simulink model "ProposedProblem5"  (R2013a)
settings: Solver=ode45  StartTime=0.0  StopTime=3600  RelTol=1e-3
undefined symbols (not defined in the file): des, gcbh
settings Model: Creator=gabig  LastModifiedBy=gabig

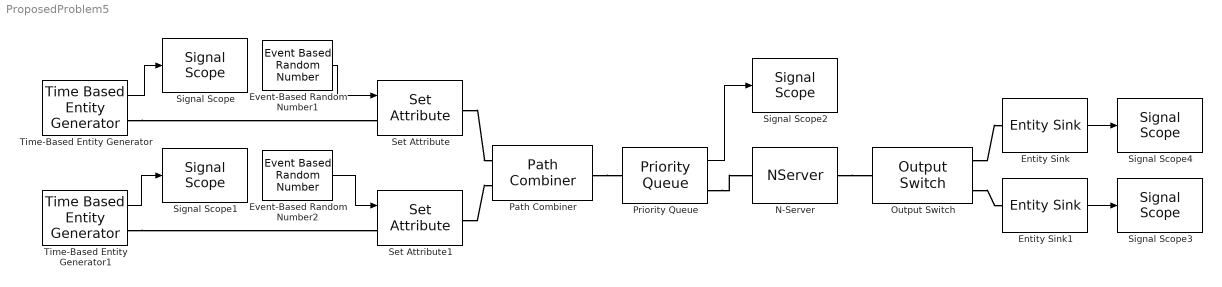
== system ProposedProblem5 ==
  Entity Sink : EntitySink  StatNumberArrived=on
  Entity Sink1 : EntitySink  StatNumberArrived=on
  Event-Based Random Number1 : EventBasedRandomNumber  Distribution=Uniform  minUnif=21  maxUnif=39  Seed=12321
  Event-Based Random Number2 : EventBasedRandomNumber  Distribution=Uniform  minUnif=9  maxUnif=15  Seed=12312
  N-Server : NServer  NumberOfServers=2  ServiceTimeFrom=Attribute  AttributeName=WORKER
  Output Switch : OutputSwitch  NumberOutputPorts=2  SwitchingCriterion=From attribute  AttributeName=p1
  Path Combiner : PathCombiner  NumberInputPorts=2
  Priority Queue : PriorityQueue  SortingAttributeName=p1  SortingDirection=Descending  StatAverageQueueLength=on
      settings: OutputPortMap=o3
  Set Attribute : SetAttribute  AttributeName=WORKER|p1  AttributeFrom=Signal port|Dialog  AttributeValue=1|1  AttributeTreatAsVector=1|1  EvaluatedAttributeValue={ [];1}
  Set Attribute1 : SetAttribute  AttributeName=WORKER|p1  AttributeFrom=Signal port|Dialog  AttributeValue=1|2  AttributeTreatAsVector=1|1  EvaluatedAttributeValue={ [];2}
  Signal Scope{,1..4} (5 alike) : SignalScope  LoadFcn=des.scope.CallbackSupport('seLoadFcn',gcbh)  StartFcn=des.scope.CallbackSupport('seStartFcn',gcbh)  StopFcn=des.scope.CallbackSupport('seStopFcn',gcbh)
      settings: CopyFcn=des.scope.CallbackSupport('seCopyFcn',gcbh)  DeleteFcn=des.scope.CallbackSupport('seDeleteFcn',gcbh)  PreSaveFcn=des.scope.CallbackSupport('sePreSaveFcn',gcbh)  NameChangeFcn=des.scope.CallbackSupport('seNameChangeFcn',gcbh)  OpenFcn=des.scope.CallbackSupport('seOpenFcn',gcbh)
  Time-Based Entity Generator : TimeBasedEntityGenerator  Distribution=Uniform  InitialSeed=12343  Minimum=39  Maximum=45  StatNumberDeparted=on
  Time-Based Entity Generator1 : TimeBasedEntityGenerator  Distribution=Uniform  InitialSeed=12341  Minimum=40  Maximum=60  StatNumberDeparted=on
  wires:
  Time-Based Entity Generator/1 -> Signal Scope/1
  Time-Based Entity Generator1/1 -> Signal Scope1/1
  Entity Sink1/1 -> Signal Scope3/1
  Entity Sink/1 -> Signal Scope4/1
  Event-Based Random Number1/1 -> Set Attribute/1
  Event-Based Random Number2/1 -> Set Attribute1/1
  Priority Queue/1 -> Signal Scope2/1
  connections:
  Time-Based Entity Generator1/RConn1 -- Set Attribute1/LConn1
  Priority Queue/RConn1 -- N-Server/LConn1
  Time-Based Entity Generator/RConn1 -- Set Attribute/LConn1
  Set Attribute/RConn1 -- Path Combiner/LConn1
  Output Switch/RConn2 -- Entity Sink1/LConn1
  Set Attribute1/RConn1 -- Path Combiner/LConn2
  Path Combiner/RConn1 -- Priority Queue/LConn1
  N-Server/RConn1 -- Output Switch/LConn1
  Output Switch/RConn1 -- Entity Sink/LConn1
